simulink model "first_option"  (R2020a)
settings: Solver=VariableStepAuto  StartTime=0.0  StopTime=250  RelTol=1e-3
libraries: autolibshared x1
settings Model: Creator=shiqihang  LastModifiedBy=shiqihang

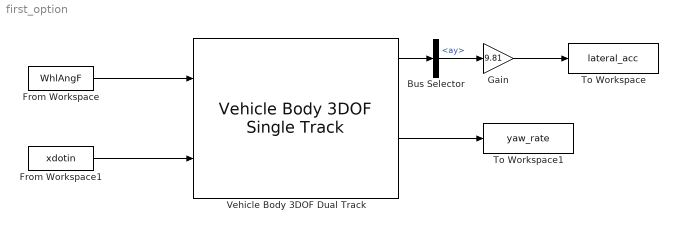
== system first_option ==
  Bus Selector : BusSelector  OutputSignals=BdyFrm.Cg.Acc.ay
  From Workspace : FromWorkspace  VariableName=WhlAngF
  From Workspace1 : FromWorkspace  VariableName=xdotin
  Gain : Gain  Gain=9.81
  To Workspace : ToWorkspace  VariableName=lateral_acc  SaveFormat=Timeseries  SampleTime=0.1
  To Workspace1 : ToWorkspace  VariableName=yaw_rate  SaveFormat=Timeseries  SampleTime=0.1
  Vehicle Body 3DOF Dual Track : autolibshared/Vehicle Body 3DOF Single Track  trackMode=Dual  inputMode=External longitudinal velocity  frontSteerMode=on  rearSteerMode=off  windMode=off  muMode=off  extFMode=off  extMMode=off  extXo=off  extpsio=off  extxdoto=off  extro=off  extYo=off  extTamb=off  extydoto=off  aMode=2  NF=2  NR=2  m=1700  a=1.5  b=1.5  h=0.35  X_o=0  xdot_o=0  CalphaMode=off  sigmaMode=on  d=0  w=[1.4,1.4]  Cy_f=29963.5  Cy_r=29963.5  sigma_f=.1  sigma_r=.1  alpha_f_brk=[-.1 .1]  Cy_f_data=[-9e3 9e3]  alpha_r_brk=[-.1 .1]  Cy_r_data=[-9e3 9e3]  Y_o=0  ydot_o=0  Izz=4000  psi_o=0  r_o=0  Af=2  Cd=.3  Cl=.1  Cpm=.1  beta_w=[0:0.01:0.3]  Cs=[0:0.03:0.9]  Cym=[0:0.01:0.3]  Pabs=101325  Tair=273  g=9.81  mu=1  xdot_tol=.01  Fznom=5000  Fxtire_sat=7e4  Fytire_sat=7e4  longOff=0  latOff=0  vertOff=0  wrapAng=off
      settings: SourceProductBaseCode=PW,MT,VE,VP
  wires:
  From Workspace/1 -> Vehicle Body 3DOF Dual Track/1
  From Workspace1/1 -> Vehicle Body 3DOF Dual Track/2
  Vehicle Body 3DOF Dual Track/1 -> Bus Selector/1
  Bus Selector/1 -> Gain/1  "<ay>"
  Vehicle Body 3DOF Dual Track/5 -> To Workspace1/1
  Gain/1 -> To Workspace/1
